simulink model "Temp_model_wk1"  (R2023b)
settings: Solver=VariableStepAuto  StartTime=0.0  StopTime=10.0  RelTol=1e-3
undefined symbols (not defined in the file): C0, C1, C2, Iw, M, rw
settings Model: Creator=kkern  LastModifiedBy=kkern

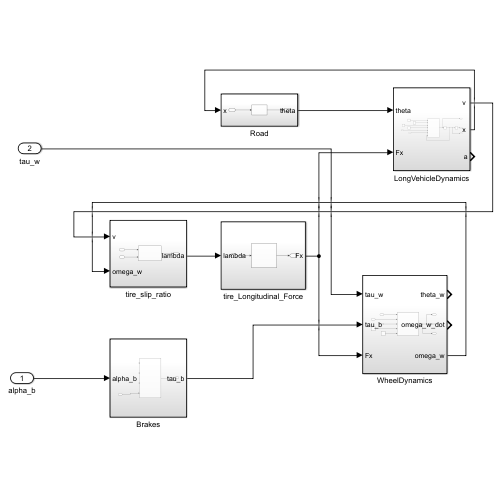
[thumbnail: Simulink's stored preview of the top-level diagram]
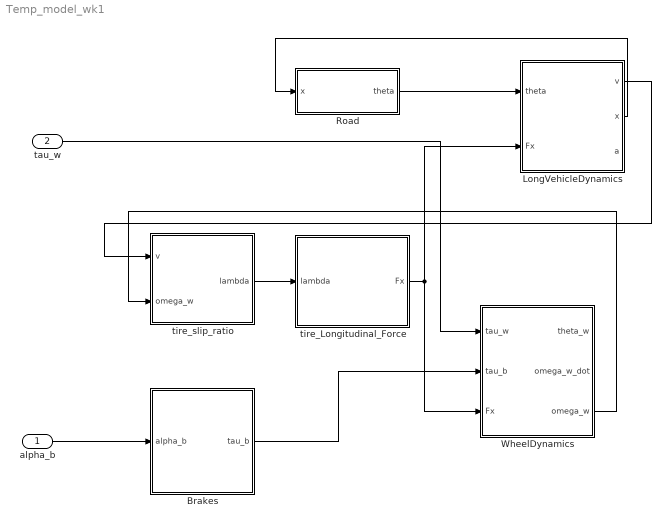
== system Temp_model_wk1 ==
  alpha_b : Inport
  tau_w : Inport  Port=2
  Brakes : Subsystem
  LongVehicleDynamics : Subsystem
  Road : Subsystem
  WheelDynamics : Subsystem
  tire_Longitudinal_Force : Subsystem
  tire_slip_ratio : Subsystem
  wires:
  tire_slip_ratio/1(lambda) -> tire_Longitudinal_Force/1(lambda)
  Road/1(theta) -> LongVehicleDynamics/1("theta ")
  LongVehicleDynamics/2("x ") -> Road/1(x)
  alpha_b/1 -> Brakes/1(alpha_b)
  tau_w/1 -> WheelDynamics/1(tau_w)
  tire_Longitudinal_Force/1(Fx) -> WheelDynamics/3(Fx), LongVehicleDynamics/2("Fx ")
  Brakes/1(tau_b) -> WheelDynamics/2(tau_b)
  WheelDynamics/3(omega_w) -> tire_slip_ratio/2(omega_w)
  LongVehicleDynamics/1("v ") -> tire_slip_ratio/1(v)

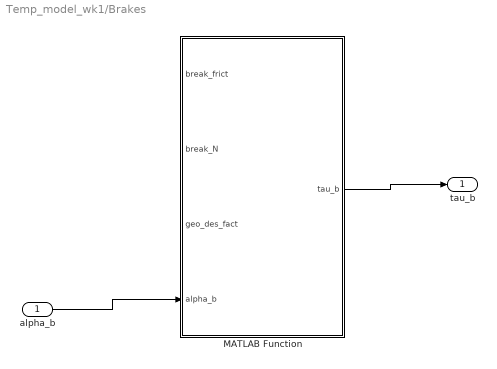
== system Temp_model_wk1/Brakes ==
  alpha_b : Inport
  MATLAB Function : MATLAB Function  TreatAsAtomicUnit=on
  tau_b : Outport
  wires:
  MATLAB Function/1(tau_b) -> tau_b/1
  alpha_b/1 -> MATLAB Function/4(alpha_b)

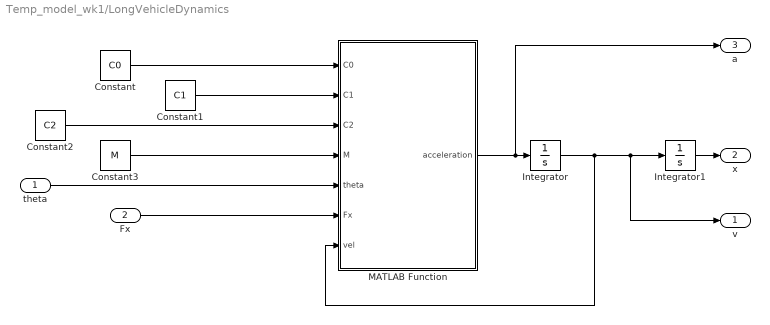
== system Temp_model_wk1/LongVehicleDynamics ==
  "theta " : Inport
  "Fx " : Inport  Port=2
  Constant : Constant  Value=C0
  Constant1 : Constant  Value=C1
  Constant2 : Constant  Value=C2
  Constant3 : Constant  Value=M
  Integrator : Integrator  LimitOutput=on  LowerSaturationLimit=0
  Integrator1 : Integrator
  MATLAB Function : MATLAB Function  TreatAsAtomicUnit=on
  "v " : Outport  VectorParamsAs1DForOutWhenUnconnected=off
  "x " : Outport  Port=2  VectorParamsAs1DForOutWhenUnconnected=off
  a : Outport  Port=3
  wires:
  Integrator1/1 -> "x "/1
  "theta "/1 -> MATLAB Function/5(theta)
  "Fx "/1 -> MATLAB Function/6(Fx)
  Constant1/1 -> MATLAB Function/2(C1)
  Constant3/1 -> MATLAB Function/4(M)
  MATLAB Function/1(acceleration) -> a/1, Integrator/1
  Constant2/1 -> MATLAB Function/3(C2)
  Integrator/1 -> MATLAB Function/7(vel), "v "/1, Integrator1/1
  Constant/1 -> MATLAB Function/1(C0)

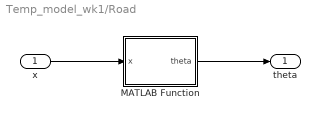
== system Temp_model_wk1/Road ==
  x : Inport
  MATLAB Function : MATLAB Function  TreatAsAtomicUnit=on
  theta : Outport
  wires:
  x/1 -> MATLAB Function/1(x)
  MATLAB Function/1(theta) -> theta/1

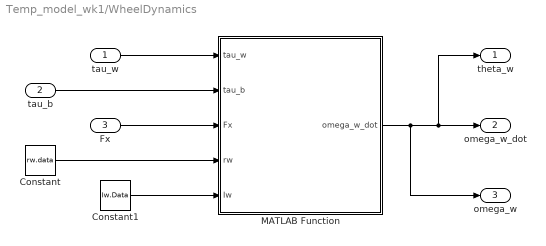
== system Temp_model_wk1/WheelDynamics ==
  tau_w : Inport
  tau_b : Inport  Port=2
  Fx : Inport  Port=3
  Constant : Constant  Value=rw.data
  Constant1 : Constant  Value=Iw.Data
  MATLAB Function : MATLAB Function  TreatAsAtomicUnit=on
  theta_w : Outport
  omega_w_dot : Outport  Port=2
  omega_w : Outport  Port=3
  wires:
  tau_w/1 -> MATLAB Function/1(tau_w)
  tau_b/1 -> MATLAB Function/2(tau_b)
  Fx/1 -> MATLAB Function/3(Fx)
  Constant1/1 -> MATLAB Function/5(Iw)
  Constant/1 -> MATLAB Function/4(rw)
  MATLAB Function/1(omega_w_dot) -> omega_w/1, theta_w/1, omega_w_dot/1

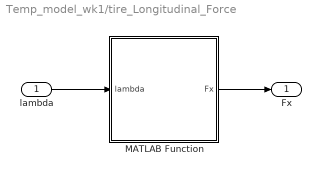
== system Temp_model_wk1/tire_Longitudinal_Force ==
  lambda : Inport
  MATLAB Function : MATLAB Function  TreatAsAtomicUnit=on
  Fx : Outport
  wires:
  lambda/1 -> MATLAB Function/1(lambda)
  MATLAB Function/1(Fx) -> Fx/1

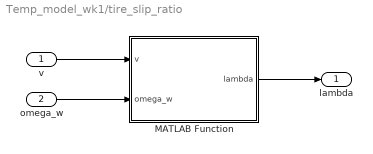
== system Temp_model_wk1/tire_slip_ratio ==
  v : Inport
  omega_w : Inport  Port=2
  MATLAB Function : MATLAB Function  TreatAsAtomicUnit=on
  lambda : Outport
  wires:
  v/1 -> MATLAB Function/1(v)
  MATLAB Function/1(lambda) -> lambda/1
  omega_w/1 -> MATLAB Function/2(omega_w)

== matlab function Temp_model_wk1/WheelDynamics/MATLAB Function ==
  data: tau_w input; omega_w_dot output; tau_b input; Fx input; rw input; Iw input
function omega_w_dot = fcn(tau_w, tau_b, Fx, rw, Iw)

omega_w_dot = (tau_w - tau_b - (Fx * rw)) / Iw;

== matlab function Temp_model_wk1/Brakes/MATLAB Function ==
  data: break_frict input; tau_b output; break_N input; geo_des_fact input; alpha_b input
function tau_b = fcn(break_frict, break_N, geo_des_fact, alpha_b)

tau_b = break_frict * break_N * geo_des_fact * sin(alpha_b);

== matlab function Temp_model_wk1/tire_Longitudinal_Force/MATLAB Function ==
  data: lambda input; Fx output
function Fx = fcn(lambda)

Fx = lambda * const_lambda;

== matlab function Temp_model_wk1/tire_slip_ratio/MATLAB Function ==
  data: v input; lambda output; omega_w input
function lambda = fcn(v, omega_w)

lambda = v * omega_w;

== matlab function Temp_model_wk1/Road/MATLAB Function ==
  data: x input; theta output
function theta = fcn(x)

theta = x;

== matlab function Temp_model_wk1/LongVehicleDynamics/MATLAB Function ==
  data: C0 input; acceleration output; C1 input; C2 input; M input; theta input; Fx input; vel input
function acceleration   = vehicle(C0,C1,C2,M,theta,Fx, vel)

acceleration = (((theta-Fx))-(C0+ C1*vel + C2*(vel)^2))/(M);
